simulink model "RLFactorySensorNoise"  (R2020b)
settings: Solver=VariableStepAuto  StartTime=0.0  StopTime=10.0  RelTol=1e-3
undefined symbols (not defined in the file): BLOCKEDTIMER, CUTOFF, DMAX, GOALSA, GOALSB, INITBX, INITBY, INTERFERENCEMAX, INTERFERENCEMIN, MAXVELOA, MAXVELOB, SAFETYDISTANCEA, SAFETYDISTANCEB, THRESHOLDA, THRESHOLDB, TSA, TSB, TSRL
libraries: rllib x1
(part 2 of 2)

== system RLFactorySensorNoise/RLServiceOpponentB/RLServiceAOpponentController/RLServiceArrivedChecker/RLServiceEuclideanDistanceCalculator2 ==
  X : Inport
  Y : Inport  Port=2
  GoalX : Inport  Port=3
  GoalY : Inport  Port=4
  Square : Math  Operator=square  SaturateOnIntegerOverflow=on
  Square Root : Sqrt  SaturateOnIntegerOverflow=on
  Square1 : Math  Operator=square  SaturateOnIntegerOverflow=on
  Sum1 : Sum
  Sum3 : Sum  Inputs=+-
  Sum4 : Sum  Inputs=+-
  OppDistToGoal : Outport
  wires:
  GoalX/1 -> Sum3/2
  X/1 -> Sum3/1
  Sum1/1 -> Square Root/1
  Sum4/1 -> Square1/1
  Square/1 -> Sum1/1
  Y/1 -> Sum4/1
  Square Root/1 -> OppDistToGoal/1
  Square1/1 -> Sum1/2
  Sum3/1 -> Square/1
  GoalY/1 -> Sum4/2

== system RLFactorySensorNoise/RLServiceRLRobotNoise/RLServiceRLInfo/RLServiceCrashDetector/RLServiceEuclideanDistanceCalculator1 ==
  X : Inport
  Y : Inport  Port=2
  XOpp : Inport  Port=3
  YOpp : Inport  Port=4
  Square : Math  Operator=square  SaturateOnIntegerOverflow=on
  Square Root : Sqrt  SaturateOnIntegerOverflow=on
  Square1 : Math  Operator=square  SaturateOnIntegerOverflow=on
  Sum1 : Sum
  Sum3 : Sum  Inputs=+-
  Sum4 : Sum  Inputs=+-
  Dist : Outport
  wires:
  XOpp/1 -> Sum3/2
  X/1 -> Sum3/1
  Sum1/1 -> Square Root/1
  Sum4/1 -> Square1/1
  Square/1 -> Sum1/1
  Y/1 -> Sum4/1
  Square Root/1 -> Dist/1
  Square1/1 -> Sum1/2
  Sum3/1 -> Square/1
  YOpp/1 -> Sum4/2

== system RLFactorySensorNoise/RLServiceRLRobotNoise/RLServiceRLInfo/RLServiceCrashDetector/RLServiceEuclideanDistanceCalculator2 ==
  X : Inport
  Y : Inport  Port=2
  XOpp : Inport  Port=3
  YOpp : Inport  Port=4
  Square : Math  Operator=square  SaturateOnIntegerOverflow=on
  Square Root : Sqrt  SaturateOnIntegerOverflow=on
  Square1 : Math  Operator=square  SaturateOnIntegerOverflow=on
  Sum1 : Sum
  Sum3 : Sum  Inputs=+-
  Sum4 : Sum  Inputs=+-
  Dist : Outport
  wires:
  XOpp/1 -> Sum3/2
  X/1 -> Sum3/1
  Sum1/1 -> Square Root/1
  Sum4/1 -> Square1/1
  Square/1 -> Sum1/1
  Y/1 -> Sum4/1
  Square Root/1 -> Dist/1
  Square1/1 -> Sum1/2
  Sum3/1 -> Square/1
  YOpp/1 -> Sum4/2

== system RLFactorySensorNoise/RLServiceRLRobotNoise/RLServiceRLInfo/RLServiceGoalTracker/RLServiceEuclideanDistanceCalculator ==
  X : Inport
  Y : Inport  Port=2
  GoalX : Inport  Port=3
  GoalY : Inport  Port=4
  Square : Math  Operator=square  SaturateOnIntegerOverflow=on
  Square Root : Sqrt  SaturateOnIntegerOverflow=on
  Square1 : Math  Operator=square  SaturateOnIntegerOverflow=on
  Sum1 : Sum
  Sum3 : Sum  Inputs=+-
  Sum4 : Sum  Inputs=+-
  DistGoal : Outport
  wires:
  GoalX/1 -> Sum3/2
  X/1 -> Sum3/1
  Sum1/1 -> Square Root/1
  Sum4/1 -> Square1/1
  Square/1 -> Sum1/1
  Y/1 -> Sum4/1
  Square Root/1 -> DistGoal/1
  Square1/1 -> Sum1/2
  Sum3/1 -> Square/1
  GoalY/1 -> Sum4/2

== system RLFactorySensorNoise/RLServiceRLRobotNoise/RLServiceRLRobotSensorWithDMAXAndNoise/RLServiceARobotSensorSubsystemWithDMAXAndNoise/RLServiceNoise ==
  Uniform Random Number1 : UniformRandomNumber  Minimum=INTERFERENCEMIN  Maximum=INTERFERENCEMAX  SampleTime=0.1
  Out1 : Outport
  wires:
  Uniform Random Number1/1 -> Out1/1

== system RLFactorySensorNoise/RLServiceRLRobotNoise/RLServiceRLRobotSensorWithDMAXAndNoise/RLServiceARobotSensorSubsystemWithDMAXAndNoise/RLServiceRobotSensorSubsystem ==
  X : Inport
  Y : Inport  Port=2
  XOpp : Inport  Port=3
  YOpp : Inport  Port=4
  Demux4 : Demux  Outputs=2
  Demux6 : Demux  Outputs=2
  Mux : Mux  Inputs=2
  Mux1 : Mux  Inputs=2
  RLServiceDirectionCalculator : Subsystem
  Sum : Sum  Inputs=-+|
  DiffXOpp : Outport
  DiffYOpp : Outport  Port=2
  DirXOpp : Outport  Port=3
  DirYOpp : Outport  Port=4
  wires:
  Mux/1 -> Sum/2, Demux6/1
  Demux6/2 -> RLServiceDirectionCalculator/2(OppY)
  XOpp/1 -> Mux/1
  X/1 -> Mux1/1
  Y/1 -> Mux1/2
  Demux6/1 -> RLServiceDirectionCalculator/1(OppX)
  RLServiceDirectionCalculator/1(DirOppX) -> DirXOpp/1
  YOpp/1 -> Mux/2
  Mux1/1 -> Sum/1
  Sum/1 -> Demux4/1
  RLServiceDirectionCalculator/2(DirOppY) -> DirYOpp/1
  Demux4/2 -> DiffYOpp/1
  Demux4/1 -> DiffXOpp/1

== system RLFactorySensorNoise/RLServiceRLRobotNoise/RLServiceRLRobotSensorWithDMAXAndNoise/RLServiceBRobotSensorSubsystemWithDMAXAndNoise/RLServiceNoise ==
  Uniform Random Number1 : UniformRandomNumber  Minimum=INTERFERENCEMIN  Maximum=INTERFERENCEMAX  SampleTime=0.1
  Out1 : Outport
  wires:
  Uniform Random Number1/1 -> Out1/1

== system RLFactorySensorNoise/RLServiceRLRobotNoise/RLServiceRLRobotSensorWithDMAXAndNoise/RLServiceBRobotSensorSubsystemWithDMAXAndNoise/RLServiceRobotSensorSubsystem ==
  X : Inport
  Y : Inport  Port=2
  XOpp : Inport  Port=3
  YOpp : Inport  Port=4
  Demux4 : Demux  Outputs=2
  Demux6 : Demux  Outputs=2
  Mux : Mux  Inputs=2
  Mux1 : Mux  Inputs=2
  RLServiceDirectionCalculator : Subsystem
  Sum : Sum  Inputs=-+|
  DiffOppX : Outport
  DiffOppY : Outport  Port=2
  DirOppX : Outport  Port=3
  DirOppY : Outport  Port=4
  wires:
  Demux4/1 -> DiffOppX/1
  Demux4/2 -> DiffOppY/1
  RLServiceDirectionCalculator/2(DirOppY) -> DirOppY/1
  Sum/1 -> Demux4/1
  Mux1/1 -> Sum/1
  YOpp/1 -> Mux/2
  RLServiceDirectionCalculator/1(DirOppX) -> DirOppX/1
  Demux6/1 -> RLServiceDirectionCalculator/1(OppX)
  Y/1 -> Mux1/2
  X/1 -> Mux1/1
  XOpp/1 -> Mux/1
  Demux6/2 -> RLServiceDirectionCalculator/2(OppY)
  Mux/1 -> Demux6/1, Sum/2

== system RLFactorySensorNoise/RLServiceRLRobotNoise/RLServiceRLRobotSensorWithDMAXAndNoise/RLServiceARobotSensorSubsystemWithDMAXAndNoise/RLServiceRobotSensorSubsystem/RLServiceDirectionCalculator ==
  OppX : Inport
  OppY : Inport  Port=2
  Demux : Demux  Outputs=2
  Mux : Mux  Inputs=2
  Sign : Signum
  Sign1 : Signum
  Sum : Sum  Inputs=+-
  Unit Delay : UnitDelay  SampleTime=TSRL  HasFrameUpgradeWarning=on
  DirOppX : Outport
  DirOppY : Outport  Port=2
  wires:
  Mux/1 -> Unit Delay/1, Sum/1
  Unit Delay/1 -> Sum/2
  Sum/1 -> Demux/1
  Demux/1 -> Sign1/1
  Demux/2 -> Sign/1
  Sign1/1 -> DirOppX/1
  Sign/1 -> DirOppY/1
  OppX/1 -> Mux/1
  OppY/1 -> Mux/2

== system RLFactorySensorNoise/RLServiceRLRobotNoise/RLServiceRLRobotSensorWithDMAXAndNoise/RLServiceBRobotSensorSubsystemWithDMAXAndNoise/RLServiceRobotSensorSubsystem/RLServiceDirectionCalculator ==
  OppX : Inport
  OppY : Inport  Port=2
  Demux : Demux  Outputs=2
  Mux : Mux  Inputs=2
  Sign : Signum
  Sign1 : Signum
  Sum : Sum  Inputs=+-
  Unit Delay : UnitDelay  SampleTime=TSRL  HasFrameUpgradeWarning=on
  DirOppX : Outport
  DirOppY : Outport  Port=2
  wires:
  OppY/1 -> Mux/2
  OppX/1 -> Mux/1
  Sign/1 -> DirOppY/1
  Sign1/1 -> DirOppX/1
  Demux/2 -> Sign/1
  Demux/1 -> Sign1/1
  Sum/1 -> Demux/1
  Unit Delay/1 -> Sum/2
  Mux/1 -> Sum/1, Unit Delay/1
